simulink model "thirdSimulinkQuestion"  (R2020b)
settings: Solver=VariableStepAuto  StartTime=0.0  StopTime=10  RelTol=1e-3
settings Model: Creator=parke  LastModifiedBy=parke

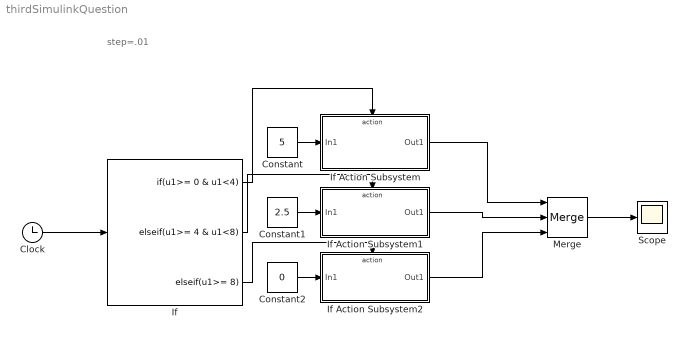
== system thirdSimulinkQuestion ==
  note: step=.01
  Clock : Clock
  Constant : Constant  Value=5
  Constant1 : Constant  Value=2.5
  Constant2 : Constant  Value=0
  If : If  IfExpression=u1>= 0 & u1<4  ElseIfExpressions=u1>= 4 & u1<8, u1>= 8  ShowElse=off
  If Action Subsystem : Subsystem  TreatAsAtomicUnit=on
  If Action Subsystem1 : Subsystem  TreatAsAtomicUnit=on
  If Action Subsystem2 : Subsystem  TreatAsAtomicUnit=on
  Merge : Merge  Inputs=3
  Scope : Scope
  wires:
  Clock/1 -> If/1
  Merge/1 -> Scope/1
  If/1 -> If Action Subsystem/Action
  If/2 -> If Action Subsystem1/Action
  If/3 -> If Action Subsystem2/Action
  Constant/1 -> If Action Subsystem/1(In1)
  Constant1/1 -> If Action Subsystem1/1(In1)
  Constant2/1 -> If Action Subsystem2/1(In1)
  If Action Subsystem2/1(Out1) -> Merge/3
  If Action Subsystem1/1(Out1) -> Merge/2
  If Action Subsystem/1(Out1) -> Merge/1

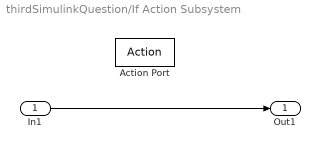
== system thirdSimulinkQuestion/If Action Subsystem ==
  In1 : Inport
  Action Port : ActionPort  ActionPortLabel=if(u1>= 0 & u1<4)
  Out1 : Outport
  wires:
  In1/1 -> Out1/1

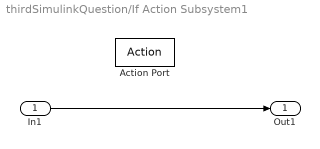
== system thirdSimulinkQuestion/If Action Subsystem1 ==
  In1 : Inport
  Action Port : ActionPort  ActionPortLabel=elseif(u1>= 4 & u1<8)
  Out1 : Outport
  wires:
  In1/1 -> Out1/1

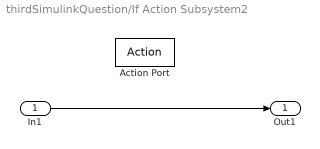
== system thirdSimulinkQuestion/If Action Subsystem2 ==
  In1 : Inport
  Action Port : ActionPort  ActionPortLabel=elseif( u1>= 8)
  Out1 : Outport
  wires:
  In1/1 -> Out1/1
